simulink model "prob8_214869"  (R2020a)
settings: Solver=VariableStepAuto  StartTime=0.0  StopTime=10.0  RelTol=1e-3
libraries: sf_elevator_lib x1
settings Model: Creator=sonal  LastModifiedBy=sonal

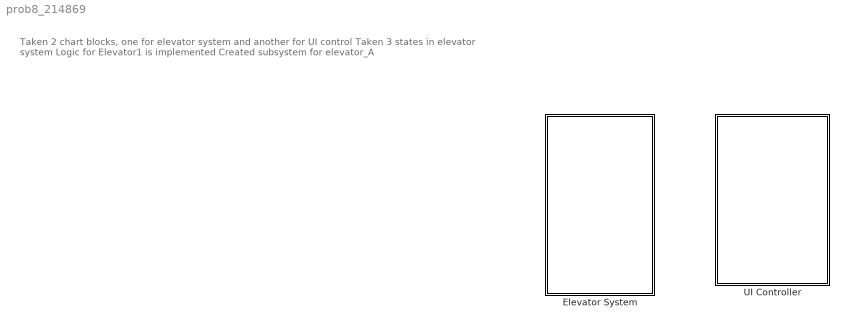
== system prob8_214869 ==
  note: Taken 2 chart blocks, one for elevator system and another for UI control
      | Taken 3 states in elevator system
      | Logic for Elevator1 is implemented
      | Created subsystem for elevator_A
  Elevator System : Stateflow chart  TreatAsAtomicUnit=on
  UI Controller : Stateflow chart  TreatAsAtomicUnit=on

== stateflow chart prob8_214869/Elevator System ==
  state Elevator_A1

== stateflow chart prob8_214869/UI Controller ==
